simulink model "AssistTrajectory"  (R2024b)
settings: Solver=ode45  StartTime=0.0  StopTime=33.66  FixedStep=.001  MaxStep=0.001  RelTol=1e-1
libraries: simulink x3
settings Model: Creator=hjhje  LastModifiedBy=hjhje

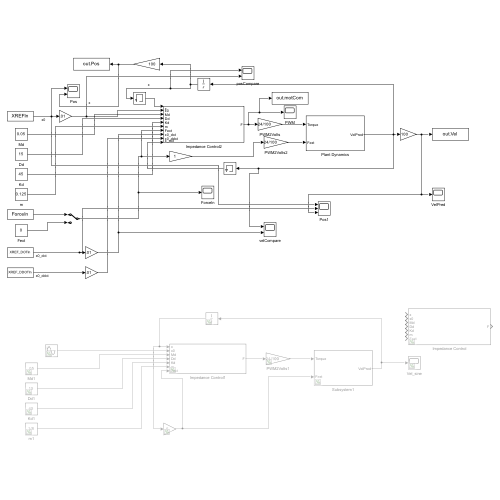
[thumbnail: Simulink's stored preview of the top-level diagram]
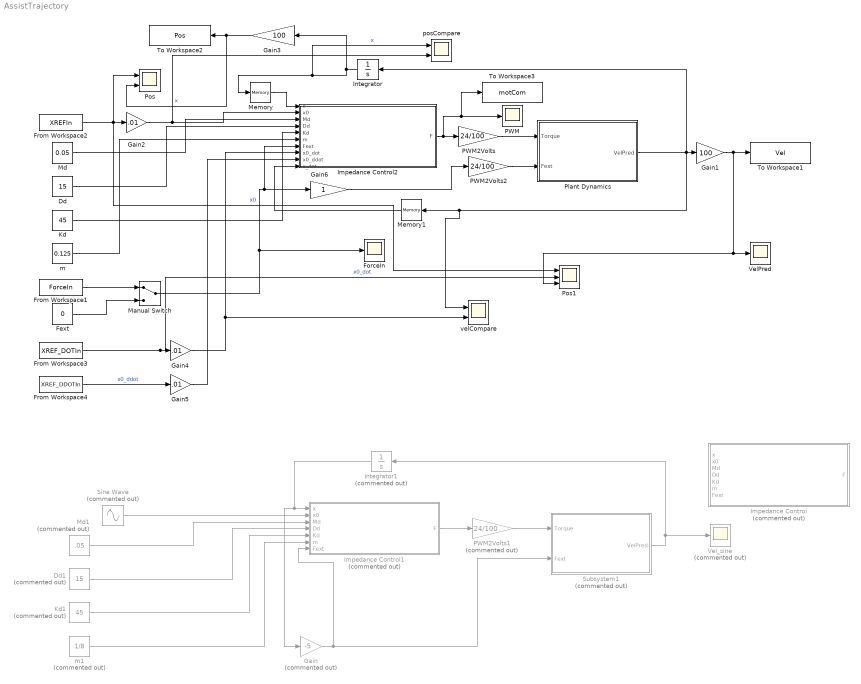
== system AssistTrajectory ==
  Dd : Constant  Value=15
  Dd1 : Constant  Commented=on  Value=15
  Fext : Constant  Value=0
  ForceIn : Scope
  From Workspace1 : FromWorkspace  VariableName=ForceIn  SampleTime=-1  Interpolate=off  OutputAfterFinalValue=Holding final value
  From Workspace2 : FromWorkspace  VariableName=XREFIn  SampleTime=-1  Interpolate=off  OutputAfterFinalValue=Holding final value
  From Workspace3 : FromWorkspace  VariableName=XREF_DOTIn  SampleTime=-1  Interpolate=off  OutputAfterFinalValue=Holding final value
  From Workspace4 : FromWorkspace  VariableName=XREF_DDOTIn  SampleTime=-1  Interpolate=off  OutputAfterFinalValue=Holding final value
  Gain : Gain  Commented=on  Gain=-5
  Gain1 : Gain  Gain=100
  Gain2 : Gain  Gain=.01
  Gain3 : Gain  Gain=100
  Gain4 : Gain  Gain=.01
  Gain5 : Gain  Gain=.01
  Gain6 : Gain
  Impedance Control : Subsystem  Commented=on
  Impedance Control1 : Subsystem  Commented=on
  Impedance Control2 : Subsystem
  Integrator : Integrator
  Integrator1 : Integrator  Commented=on
  Kd : Constant  Value=45
  Kd1 : Constant  Commented=on  Value=45
  Manual Switch : ManualSwitch
  Md : Constant  Value=0.05
  Md1 : Constant  Commented=on  Value=.05
  Memory : Memory
  Memory1 : Memory
  PWM : Scope
  PWM2Volts : Gain  Gain=24/100
  PWM2Volts1 : Gain  Commented=on  Gain=24/100
  PWM2Volts2 : Gain  Gain=24/100
  Plant Dynamics : Subsystem
  Pos : Scope  NumInputPorts=2
  Pos1 : Scope  NumInputPorts=3
  Sine Wave : Sin  Commented=on  Amplitude=.1575  Frequency=pi/5  SampleTime=0
  Subsystem1 : Subsystem  Commented=on
  To Workspace1 : ToWorkspace  VariableName=Vel  SaveFormat=Timeseries  SampleTime=-1
  To Workspace2 : ToWorkspace  VariableName=Pos  SaveFormat=Timeseries  SampleTime=-1
  To Workspace3 : ToWorkspace  VariableName=motCom  SaveFormat=Timeseries  SampleTime=-1
  VelPred : Scope
  Vel_sine : Scope  Commented=on
  m : Constant  Value=0.125
  m1 : Constant  Commented=on  Value=1/8
  posCompare : Scope  NumInputPorts=2
  velCompare : Scope  NumInputPorts=2
  wires:
  PWM2Volts/1 -> Plant Dynamics/1(Torque)
  Impedance Control2/1(F) -> To Workspace3/1, PWM/1, PWM2Volts/1
  Plant Dynamics/1(VelPred) -> velCompare/1, Memory1/1, Gain1/1, Integrator/1
  Integrator/1 -> posCompare/1, Memory/1, Gain3/1  "x"
  From Workspace2/1 -> Pos1/1, Gain2/1, Pos/1  "x0"
  Manual Switch/1 -> ForceIn/1, Gain6/1, Impedance Control2/7(Fext)
  Md/1 -> Impedance Control2/3(Md)
  Dd/1 -> Impedance Control2/4(Dd)
  Kd/1 -> Impedance Control2/5(Kd)
  m/1 -> Impedance Control2/6(m)
  Integrator1/1 -> Gain/1, Impedance Control1/1(x)
  PWM2Volts1/1 -> Subsystem1/1(Torque)
  Impedance Control1/1(F) -> PWM2Volts1/1
  Subsystem1/1(VelPred) -> Vel_sine/1, Integrator1/1
  Md1/1 -> Impedance Control1/3(Md)
  Kd1/1 -> Impedance Control1/5(Kd)
  Dd1/1 -> Impedance Control1/4(Dd)
  m1/1 -> Impedance Control1/6(m)
  Gain/1 -> Subsystem1/2(Fext), Impedance Control1/7(Fext)
  Sine Wave/1 -> Impedance Control1/2(x0)
  Gain2/1 -> posCompare/2, Impedance Control2/2(x0)
  Gain1/1 -> Pos1/3, VelPred/1, To Workspace1/1
  Gain3/1 -> Pos/2, To Workspace2/1  "x"
  PWM2Volts2/1 -> Plant Dynamics/2(Fext)
  From Workspace1/1 -> Manual Switch/1
  Fext/1 -> Manual Switch/2
  From Workspace3/1 -> Pos1/2, Gain4/1  "x0_dot"
  From Workspace4/1 -> Gain5/1  "x0_ddot"
  Gain4/1 -> velCompare/2, Impedance Control2/8(x0_dot)
  Gain5/1 -> Impedance Control2/9(x0_ddot)
  Memory/1 -> Impedance Control2/1(x)
  Memory1/1 -> Impedance Control2/10(x_dot)
  Gain6/1 -> PWM2Volts2/1

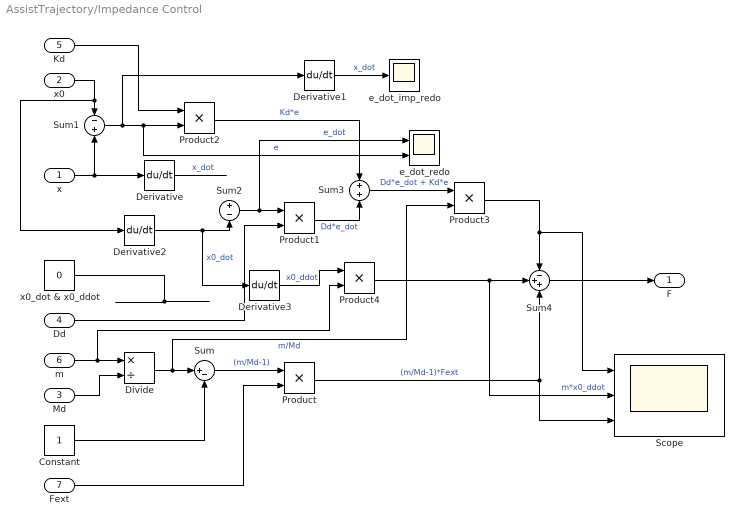
== system AssistTrajectory/Impedance Control ==
  x : Inport
  x0 : Inport  Port=2
  Md : Inport  Port=3
  Dd : Inport  Port=4
  Kd : Inport  Port=5
  m : Inport  Port=6
  Fext : Inport  Port=7
  Constant : Constant
  Derivative{,1..3} (4 alike) : Derivative
  Divide : Product  Inputs=*/
  Product{,1..4} (5 alike) : Product
  Scope : Scope  NumInputPorts=3
  Sum : Sum  Inputs=|+-
  Sum1 : Sum  Inputs=-+
  Sum2 : Sum  Inputs=+-
  Sum3 : Sum
  Sum4 : Sum  Inputs=-++
  e_dot_imp_redo : Scope
  e_dot_redo : Scope  NumInputPorts=2
  x0_dot & x0_ddot : Constant  Value=0
  F : Outport
  wires:
  m/1 -> Product4/2, Divide/1
  Md/1 -> Divide/2
  Divide/1 -> Product3/2, Sum/1  "m/Md"
  Constant/1 -> Sum/2
  Sum/1 -> Product/1  "(m/Md-1)"
  Fext/1 -> Product/2
  Product/1 -> Sum4/3, Scope/3  "(m/Md-1)*Fext"
  x/1 -> Derivative/1, Sum1/2
  Derivative/1 -> ?  "x_dot"
  Sum1/1 -> Derivative1/1, e_dot_redo/2, Product2/2  "e"
  x0_dot & x0_ddot/1 -> ?
  Sum2/1 -> e_dot_redo/1, Product1/1  "e_dot"
  x0/1 -> Derivative2/1, Sum1/1
  Dd/1 -> Product1/2
  Product1/1 -> Sum3/2  "Dd*e_dot"
  Kd/1 -> Product2/1
  Product2/1 -> Sum3/1  "Kd*e"
  Sum3/1 -> Product3/1  "Dd*e_dot + Kd*e"
  Product3/1 -> Scope/1, Sum4/1
  Sum4/1 -> F/1
  Product4/1 -> Sum4/2, Scope/2  "m*x0_ddot"
  Derivative1/1 -> e_dot_imp_redo/1  "x_dot"
  Derivative2/1 -> Derivative3/1, Sum2/2  "x0_dot"
  Derivative3/1 -> Product4/1  "x0_ddot"

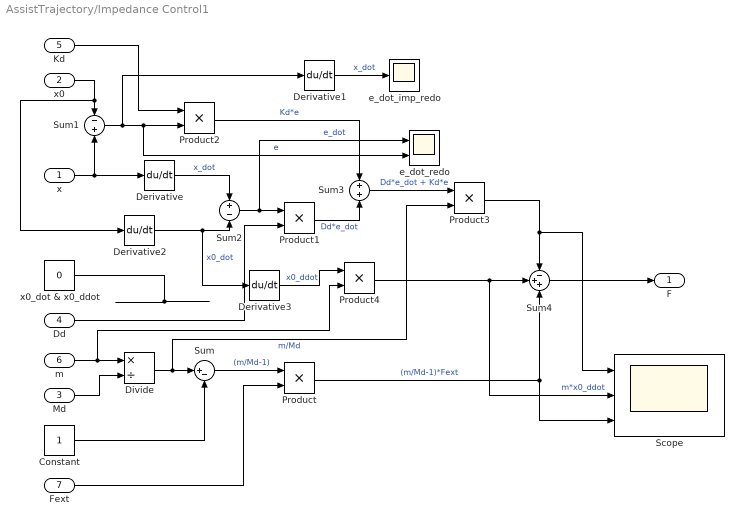
== system AssistTrajectory/Impedance Control1 ==
  x : Inport
  x0 : Inport  Port=2
  Md : Inport  Port=3
  Dd : Inport  Port=4
  Kd : Inport  Port=5
  m : Inport  Port=6
  Fext : Inport  Port=7
  Constant : Constant
  Derivative{,1..3} (4 alike) : Derivative
  Divide : Product  Inputs=*/
  Product{,1..4} (5 alike) : Product
  Scope : Scope  NumInputPorts=3
  Sum : Sum  Inputs=|+-
  Sum1 : Sum  Inputs=-+
  Sum2 : Sum  Inputs=+-
  Sum3 : Sum
  Sum4 : Sum  Inputs=-++
  e_dot_imp_redo : Scope
  e_dot_redo : Scope  NumInputPorts=2
  x0_dot & x0_ddot : Constant  Value=0
  F : Outport
  wires:
  m/1 -> Product4/2, Divide/1
  Md/1 -> Divide/2
  Divide/1 -> Product3/2, Sum/1  "m/Md"
  Constant/1 -> Sum/2
  Sum/1 -> Product/1  "(m/Md-1)"
  Fext/1 -> Product/2
  Product/1 -> Sum4/3, Scope/3  "(m/Md-1)*Fext"
  x/1 -> Derivative/1, Sum1/2
  Derivative/1 -> Sum2/1  "x_dot"
  Sum1/1 -> Derivative1/1, e_dot_redo/2, Product2/2  "e"
  x0_dot & x0_ddot/1 -> ?
  Sum2/1 -> e_dot_redo/1, Product1/1  "e_dot"
  x0/1 -> Derivative2/1, Sum1/1
  Dd/1 -> Product1/2
  Product1/1 -> Sum3/2  "Dd*e_dot"
  Kd/1 -> Product2/1
  Product2/1 -> Sum3/1  "Kd*e"
  Sum3/1 -> Product3/1  "Dd*e_dot + Kd*e"
  Product3/1 -> Scope/1, Sum4/1
  Sum4/1 -> F/1
  Product4/1 -> Sum4/2, Scope/2  "m*x0_ddot"
  Derivative1/1 -> e_dot_imp_redo/1  "x_dot"
  Derivative2/1 -> Derivative3/1, Sum2/2  "x0_dot"
  Derivative3/1 -> Product4/1  "x0_ddot"

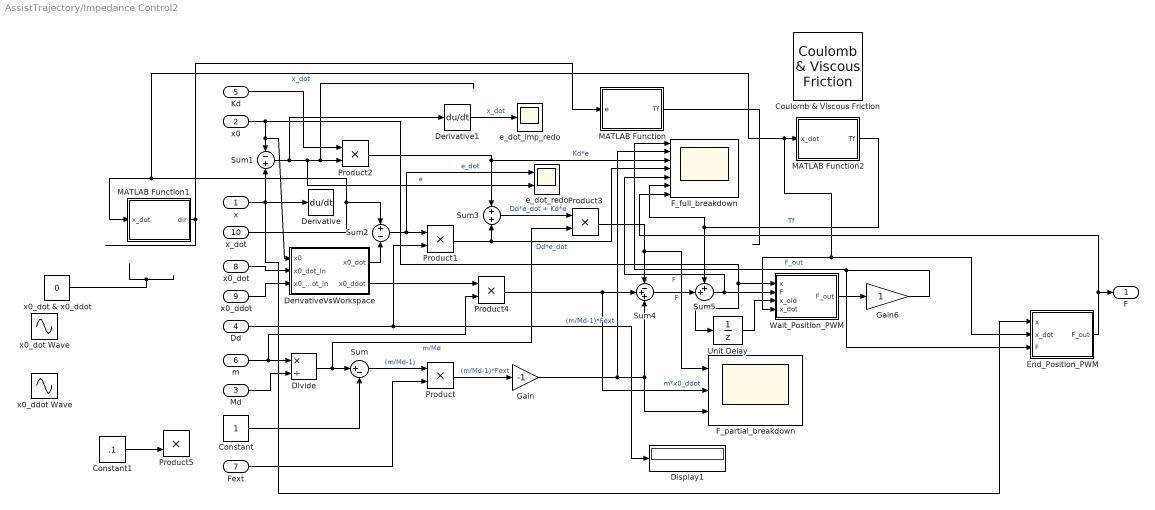
== system AssistTrajectory/Impedance Control2 ==
  x : Inport
  x0 : Inport  Port=2
  Md : Inport  Port=3
  Dd : Inport  Port=4
  Kd : Inport  Port=5
  m : Inport  Port=6
  Fext : Inport  Port=7
  x0_dot : Inport  Port=8
  x0_ddot : Inport  Port=9
  x_dot : Inport  Port=10
  Constant : Constant
  Constant1 : Constant  Value=.1
  Coulomb & Viscous Friction : simulink/Discontinuities/Coulomb & Viscous Friction  offset=10.95  gain=(1.0 / 0.090977)* (100.0 / 24.0)
  Derivative : Derivative
  Derivative1 : Derivative
  DerivativeVsWorkspace : Subsystem
  Display1 : Display
  Divide : Product  Inputs=*/
  End_Position_PWM : MATLAB Function  TreatAsAtomicUnit=on
  F_full_breakdown : Scope  NumInputPorts=7
  F_partial_breakdown : Scope  NumInputPorts=3
  Gain : Gain  Gain=-1
  Gain6 : Gain
  MATLAB Function : MATLAB Function  TreatAsAtomicUnit=on
  MATLAB Function1 : MATLAB Function  TreatAsAtomicUnit=on
  MATLAB Function2 : MATLAB Function  TreatAsAtomicUnit=on
  Product{,1..5} (6 alike) : Product
  Sum : Sum  Inputs=|+-
  Sum1 : Sum  Inputs=-+
  Sum2 : Sum  Inputs=+-
  Sum3 : Sum
  Sum4 : Sum  Inputs=-++
  Sum5 : Sum  Inputs=++|
  Unit Delay : UnitDelay  SampleTime=-1  HasFrameUpgradeWarning=on
  Wait_Position_PWM : MATLAB Function  TreatAsAtomicUnit=on
  e_dot_imp_redo : Scope
  e_dot_redo : Scope  NumInputPorts=2
  x0_ddot Wave : Sin  Amplitude=.1575*(pi/5)*(pi/5)  Frequency=pi/5  Phase=-pi/2  SampleTime=0
  x0_dot & x0_ddot : Constant  Value=0
  x0_dot Wave : Sin  Amplitude=.1575*pi/5  Frequency=pi/5  SampleTime=0
  F : Outport
  wires:
  m/1 -> Product4/2, Divide/1
  Md/1 -> Divide/2
  Divide/1 -> Product3/2, Sum/1  "m/Md"
  Constant/1 -> Sum/2
  Sum/1 -> Product/1  "(m/Md-1)"
  Fext/1 -> Product/2
  Product/1 -> Gain/1  "(m/Md-1)*Fext"
  x/1 -> End_Position_PWM/1(x), Sum1/2, Derivative/1
  x_dot/1 -> End_Position_PWM/2(x_dot), Wait_Position_PWM/4(x_dot), MATLAB Function2/1(x_dot), MATLAB Function1/1(x_dot), Sum2/1  "x_dot"
  Sum1/1 -> Derivative1/1, e_dot_redo/2, Product2/2  "e"
  x0_dot & x0_ddot/1 -> ?
  Sum2/1 -> e_dot_redo/1, Product1/1  "e_dot"
  x0/1 -> Unit Delay/1, Wait_Position_PWM/1(x), DerivativeVsWorkspace/1(x0), Sum1/1
  Dd/1 -> Display1/1, Product1/2
  Product1/1 -> F_full_breakdown/4, Sum3/2  "Dd*e_dot"
  Kd/1 -> Product2/1
  Product2/1 -> Sum3/1, F_full_breakdown/3  "Kd*e"
  Sum3/1 -> Product3/1  "Dd*e_dot + Kd*e"
  Product3/1 -> F_partial_breakdown/1, Sum4/1
  Sum5/1 -> F_full_breakdown/5, Wait_Position_PWM/2(F)  "F"
  Product4/1 -> Sum4/2, F_partial_breakdown/2  "m*x0_ddot"
  Derivative1/1 -> e_dot_imp_redo/1  "x_dot"
  Sum4/1 -> Sum5/2  "F"
  MATLAB Function/1(Tf) -> ?
  Constant1/1 -> Product5/2
  MATLAB Function1/1(dir) -> MATLAB Function/1(e)
  DerivativeVsWorkspace/1(x0_dot) -> Sum2/2
  DerivativeVsWorkspace/2(x0_ddot) -> Product4/1
  x0_dot/1 -> DerivativeVsWorkspace/2(x0_dot_In)
  x0_ddot/1 -> DerivativeVsWorkspace/3(x0_ddot_In)
  MATLAB Function2/1(Tf) -> F_full_breakdown/6, Sum5/1  "Tf"
  Gain/1 -> F_full_breakdown/2, Sum4/3, F_partial_breakdown/3  "(m/Md-1)*Fext"
  Gain6/1 -> F_full_breakdown/1, End_Position_PWM/3(F)  "F_out"
  Wait_Position_PWM/1(F_out) -> Gain6/1
  Unit Delay/1 -> Wait_Position_PWM/3(x_old)
  End_Position_PWM/1(F_out) -> F_full_breakdown/7, F/1

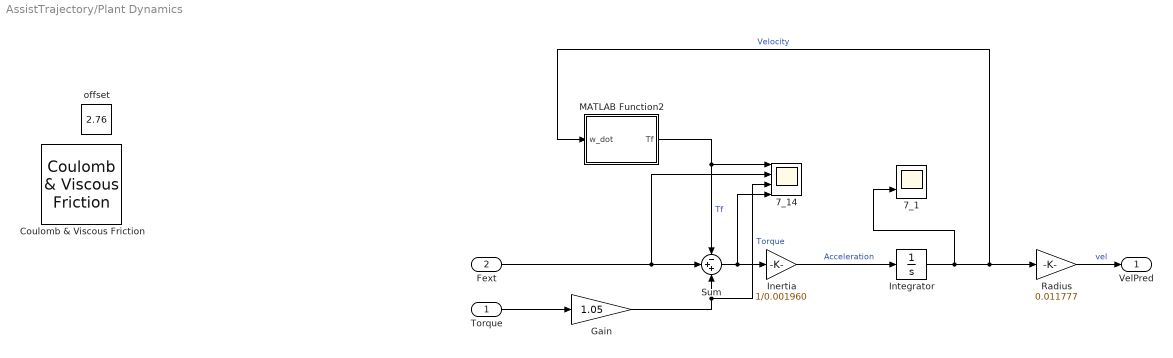
== system AssistTrajectory/Plant Dynamics ==
  Torque : Inport
  Fext : Inport  Port=2
  7_1 : Scope  NumInputPorts=2
  7_14 : Scope  NumInputPorts=4
  Coulomb & Viscous Friction : simulink/Discontinuities/Coulomb & Viscous Friction  offset=10.95*24/100  gain=1/0.090977
  Gain : Gain  Gain=1.05
  Inertia : Gain  Gain=1/0.001960
  Integrator : Integrator
  MATLAB Function2 : MATLAB Function  TreatAsAtomicUnit=on
  Radius : Gain  Gain=0.011777
  Sum : Sum  Inputs=-++
  offset : Constant  Value=2.76
  VelPred : Outport
  wires:
  Inertia/1 -> Integrator/1  "Acceleration"
  Sum/1 -> 7_14/4, Inertia/1
  MATLAB Function2/1(Tf) -> 7_14/1, Sum/1  "Tf"
  Integrator/1 -> Radius/1, MATLAB Function2/1(w_dot), 7_1/2  "Velocity"
  Torque/1 -> Gain/1
  Fext/1 -> 7_14/2, Sum/2
  Radius/1 -> VelPred/1  "vel"
  Gain/1 -> 7_14/3, Sum/3  "Torque"

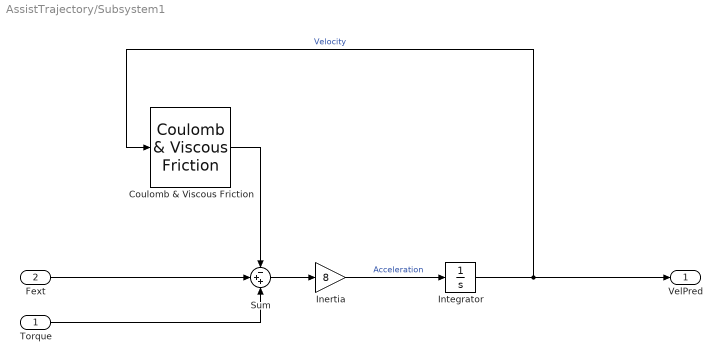
== system AssistTrajectory/Subsystem1 ==
  Torque : Inport
  Fext : Inport  Port=2
  Coulomb & Viscous Friction : simulink/Discontinuities/Coulomb & Viscous Friction  offset=2.76  gain=1/0.090977
  Inertia : Gain  Gain=8
  Integrator : Integrator
  Sum : Sum  Inputs=-++
  VelPred : Outport
  wires:
  Inertia/1 -> Integrator/1  "Acceleration"
  Sum/1 -> Inertia/1
  Coulomb & Viscous Friction/1 -> Sum/1
  Integrator/1 -> Coulomb & Viscous Friction/1, VelPred/1  "Velocity"
  Torque/1 -> Sum/3
  Fext/1 -> Sum/2

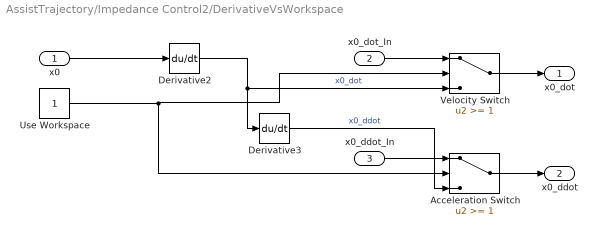
== system AssistTrajectory/Impedance Control2/DerivativeVsWorkspace ==
  x0 : Inport
  x0_dot_In : Inport  Port=2
  x0_ddot_In : Inport  Port=3
  Acceleration Switch : Switch  Threshold=1  SaturateOnIntegerOverflow=off  InputSameDT=off
  Derivative2 : Derivative
  Derivative3 : Derivative
  Use Workspace : Constant
  Velocity Switch : Switch  Threshold=1  SaturateOnIntegerOverflow=off  InputSameDT=off
  x0_dot : Outport
  x0_ddot : Outport  Port=2
  wires:
  Derivative2/1 -> Velocity Switch/3, Derivative3/1  "x0_dot"
  Derivative3/1 -> Acceleration Switch/3  "x0_ddot"
  x0/1 -> Derivative2/1
  Velocity Switch/1 -> x0_dot/1
  Acceleration Switch/1 -> x0_ddot/1
  Use Workspace/1 -> Acceleration Switch/2, Velocity Switch/2
  x0_dot_In/1 -> Velocity Switch/1
  x0_ddot_In/1 -> Acceleration Switch/1

== matlab function AssistTrajectory/Impedance Control2/MATLAB Function ==
  data: e input; Tf output
function Tf = fcn(e)

if (e > 0)
    dir = 1;
else
    dir = -1;
end
Tf = dir*10.95;

== matlab function AssistTrajectory/Impedance Control2/MATLAB Function1 ==
  data: x_dot input; dir output
function dir = fcn(x_dot)

dir = 0;
if (x_dot > 0)
    dir = 1;
else
    dir = -1;
end

== matlab function AssistTrajectory/Impedance Control2/MATLAB Function2 ==
  data: x_dot input; Tf output
function Tf = fcn(x_dot)

dir = 1;
viscousGain = (1.0 / 0.090977)* (100.0 / 24.0);
viscousGain = 0.1163 *100/24;
if x_dot > 0
    dir = 1;
elseif x_dot < 0
    dir = -1;
end
Tf = viscousGain*x_dot + 10.95*tanh(100*x_dot);

== matlab function AssistTrajectory/Plant Dynamics/MATLAB Function2 ==
  data: w_dot input; Tf output
function Tf = fcn(w_dot)

% viscousGain = 1.5*(1.0 / 0.090977);
viscousGain = 1.65*0.1163;
Tf = viscousGain*w_dot + 10.95*(24/100)*tanh(150*w_dot);

% 1.5*(1.0 / 0.090977) = 16.4877

== matlab function AssistTrajectory/Impedance Control2/Wait_Position_PWM ==
  data: x input; F input; F_out output; x_old input; x_dot input

function F_out = fcn(x, F, x_old, x_dot)

limitForce = 02;
% dir = 0;
% 
% if (x >= x_old)
%     if (F >= 0)
%         dir = 1;
%     else
%         dir = 0;
%     end
% else
%     if(F <= 0)
%         dir = 1;
%     else
%         dir = 0;
%     end
% end
% dir = 1;
F_out = F;
% dir = 0;
if (x > x_old)
    dir = 1;
elseif (x < x_old)
    dir = -1;
else
    
    dir = sign(x_dot); 
end
% if (x >= 0)
%     dir = 1;
% elseif (x < 0)
%     dir = -1;
% end

% if (x_dot > 0)
%     dir = 1;
% elseif(x_dot < 0)
%     dir = -1;
% end
if (abs(F) < 0.01)
    F_out = 0;
else
    if (dir == 1 && F < -limitForce)
        F_out = 2;
    elseif (dir == -1 && F > limitForce)
        F_out = -2;
    end
end

== matlab function AssistTrajectory/Impedance Control2/End_Position_PWM ==
  data: x input; x_dot input; F input; F_out output
function F_out = fcn(x, x_dot, F)

dir = 1;

if (x >= (31.5/100) && x_dot > 0)
    dir = 0;
elseif (x <= (-0.5/100) && x_dot < 0)
    dir = 0;
end
dir = 1;
F_out = dir * F;
